simulink model "CAVE_MachE_sil_test_v2"  (R2019b)
settings: configuration reference "ConfigSetDesktopFixedStep" (kept outside this file)
PreLoadFcn:
  | VSS_BICYCLE=Simulink.Variant('Dual=0');
  | VSS_DUAL=Simulink.Variant('Dual=1');
  | Dual=1;
  | load('DriveCycle2.mat')
PostLoadFcn:
  | %if any(exist('dsrtsu_mdlpostloadfcn', 'file') ~= 0), dsrtsu_mdlpostloadfcn('Execute', bdroot); end
InitFcn:
  | , if any(exist('dsmpb_private', 'file') ~= 0), dsmpb_private('dsmpb_mdlclblib', 'Init', bdroot); end,
  | load('DriveCycle2.mat')
model workspace (MAT data in the model file):
  Gas = 0.383333333333
values from neighbouring files (symbols this model uses):
  TestScnrioCycleNum = obj.getParamValue('TestScnrioCycleNum')    [ExpRefBlkCtrl.m]
undefined symbols (not defined in the file or in its folder): AccelCmd, ActTqLF_Nm_, ActTqLR_Nm_, ActTqRF_Nm_, ActTqRR_Nm_, BattChargeLimitMaxPwr, BattChargeLimitSocBpts, BattChargeLimitTbl, BattChrgCapcty, BattDischargeLimitSocBpts, BattDischargeLimitTbl, BattDischargeMaxPwr, BattNumCellsParallel, BattNumCellsSeries, BattOpenVoltCapBpts, BattOpenVoltTbl, BattResistSocBpts, BattResistTbl, BattResistTempBpts, BrakeMaxPrs, BrakeMaxTrq, ChassisDistCg2FrontAxle, ChassisDistCg2RearAxle, ChassisVehMass, CltchCmd, DecelCmd, DiffRatio, EnvGravCnst, EnvPrs, EnvTemp, FuelSpecificGrav, GearCmd, h, InitStates, lgSw, MtrEffSpdBpts, MtrEffTbl, MtrEffTrqBpts, MtrPwrMax, MtrTrqMax, RealSimPara, SteeringCmd, SupvsryCtrlRegenBrkCutOffTbl, SupvsryCtrlRegenSpdBpts, VEH
libraries: vehdynlibtire x8, vehdynlibsuspension x7, vehdynlibtirecommon x7, autolibshared x6, simulink x6, autolibutils x5, VsrLibWheel x4, autolibpowerinfoutils x3, sharedtransform x3, autolibbatterycommon x2, autolibsharedcoupling x2, autolibmappedmotor x2
(part 5 of 10)

== system CAVE_MachE_sil_test_v2/Vehicle Under Test/Vehicle/Vehicle Dynamics/Vehicle 14DOF/Wheels and Tires/VDBS ==
  WheelAng : Inport
  CamberAng : Inport  Port=2  Unit=rad
  AxleTrq : Inport  Port=3
  BrkPrs : Inport  Port=4
  Fz : Inport  Port=5  Unit=N
  r : Inport  Port=6
  VehVel : Inport  Port=7
  Ground Level : Inport  Port=8
  Friction : Inport  Port=9  Unit=1  PortDimensions=4
  Pressure : vehdynlibtirecommon/Constant  const=220000  numWheels=4
      settings: SourceProductName=Vehicle Dynamics Blockset  SourceProductBaseCode=VE
  Terminator : Terminator
  Tire2Veh : Subsystem
  Tires : Subsystem  VariantControlMode=Label  Variant=on  VariantControl=Variant1  LabelModeActiveChoice=0
  Veh2Tire : Subsystem
  scale factors with friction : Subsystem  mask{numWheels=4}
      mask prompts: numWheels "Number of wheels"
  Wheels : Outport  VectorParamsAs1DForOutWhenUnconnected=off
  FrntAxlF : Outport  Port=2  Unit=N  VectorParamsAs1DForOutWhenUnconnected=off
  RearAxlF : Outport  Port=3  Unit=N  VectorParamsAs1DForOutWhenUnconnected=off
  Omega : Outport  Port=4  VectorParamsAs1DForOutWhenUnconnected=off
  Mz : Outport  Port=5  Unit=N*m  VectorParamsAs1DForOutWhenUnconnected=off
  SuspWhlPz : Outport  Port=6  VectorParamsAs1DForOutWhenUnconnected=off
  SuspWhlVz : Outport  Port=7  VectorParamsAs1DForOutWhenUnconnected=off
  wires:
  Ground Level/1 -> Tires/9("Gnd ")
  Pressure/1 -> Tires/7("Press ")
  scale factors with friction/1(lambdas) -> Tires/8("lambda ")
  Fz/1 -> Tires/10("FzSusp "), Tire2Veh/2(Fz)
  AxleTrq/1 -> Veh2Tire/2(Axle)
  BrkPrs/1 -> Veh2Tire/3(Brake)
  VehVel/1 -> Veh2Tire/4(VehVel)
  Veh2Tire/1(T) -> Tires/1("DriveTorque ")
  Veh2Tire/2(P) -> Tires/2("Brake Pressure ")
  Veh2Tire/4(xdotAxle) -> Tires/4("Vx ")
  Veh2Tire/5(ydotAxle) -> Tires/5("Vy ")
  Veh2Tire/3(psidot) -> Tires/3("r ")
  Tires/1(" Wheels") -> Tire2Veh/1(Wheel)
  WheelAng/1 -> Veh2Tire/5(WheelSteer), Tire2Veh/4(WheelSteer)
  Tire2Veh/2(Omega) -> Omega/1
  Tire2Veh/3(FrntAxlF) -> FrntAxlF/1
  Tire2Veh/4(RearAxlF) -> RearAxlF/1
  Tire2Veh/5(<Mz>) -> Mz/1
  Friction/1 -> scale factors with friction/1(lamda_mu_x), scale factors with friction/2(lamda_mu_y)
  r/1 -> Veh2Tire/1(r)
  Veh2Tire/6(zdotAxle) -> Terminator/1
  Tire2Veh/6(SuspWhlPz) -> SuspWhlPz/1
  Tire2Veh/7(SuspWhlVz) -> SuspWhlVz/1
  CamberAng/1 -> Tires/6("Camber "), Tire2Veh/3(WheelCamber), Veh2Tire/6(WheelCamber)
  Tire2Veh/1(Wheels) -> Wheels/1

== system CAVE_MachE_sil_test_v2/Vehicle Under Test/Vehicle/Vehicle Dynamics/Vehicle 7DOF/Longitudinal Wheels 4DOF/Axle Forces ==
  note: 1) Add Subsystem or Model blocks as valid variant choices.
      | 2) You cannot connect blocks at this level. At simulation, connectivity is automatically
      | determined, based on the active variant and port name matching.
  F : Inport
  R : Inport  Port=2
  Bicycle : Subsystem  VariantControl=0
  Dual : Subsystem  VariantControl=1
  FrntAxlF : Outport  Unit=N  VectorParamsAs1DForOutWhenUnconnected=off
  RearAxlF : Outport  Port=2  Unit=N  VectorParamsAs1DForOutWhenUnconnected=off

== system CAVE_MachE_sil_test_v2/Vehicle Under Test/Vehicle/Vehicle Dynamics/Vehicle 7DOF/Longitudinal Wheels 4DOF/Tire2Veh ==
  Wheel : Inport
  Bus Selector7 : BusSelector  OutputSignals=Omega,Fx,Re,z,zdot,Kappa,Alpha
  Dead Zone2 : DeadZone  LowerValue=-5  UpperValue=5  ZeroCross=off  SaturateOnIntegerOverflow=on
  Demux : Demux  Outputs=[2,2]
  Re : Terminator
  Unary Minus1 : UnaryMinus
  Unary Minus2 : UnaryMinus
  zdot : Terminator
  FwF : Outport  VectorParamsAs1DForOutWhenUnconnected=off
  FwR : Outport  Port=2  VectorParamsAs1DForOutWhenUnconnected=off
  z : Outport  Port=3  VectorParamsAs1DForOutWhenUnconnected=off
  Omega : Outport  Port=4  VectorParamsAs1DForOutWhenUnconnected=off
  Kappa : Outport  Port=5  VectorParamsAs1DForOutWhenUnconnected=off
  Alpha : Outport  Port=6  VectorParamsAs1DForOutWhenUnconnected=off
  wires:
  Bus Selector7/2 -> Dead Zone2/1  "<Fx>"
  Dead Zone2/1 -> Demux/1  "Fx"
  Demux/1 -> FwF/1
  Wheel/1 -> Bus Selector7/1
  Bus Selector7/1 -> Omega/1  "<Omega>"
  Bus Selector7/5 -> Unary Minus2/1  "<zdot>"
  Bus Selector7/4 -> Unary Minus1/1  "<z>"
  Unary Minus1/1 -> z/1  "z"
  Demux/2 -> FwR/1
  Bus Selector7/6 -> Kappa/1  "<Kappa>"
  Unary Minus2/1 -> zdot/1  "zdot"
  Bus Selector7/3 -> Re/1  "<Re>"
  Bus Selector7/7 -> Alpha/1  "<Alpha>"

== system CAVE_MachE_sil_test_v2/Vehicle Under Test/Vehicle/Vehicle Dynamics/Vehicle 7DOF/Longitudinal Wheels 4DOF/Tires ==
  AxlTrq : Inport
  BrkPrs : Inport  Port=2
  Vx : Inport  Port=3
  Vy : Inport  Port=4
  r : Inport  Port=5
  Camber : Inport  Port=6
  TirePrs : Inport  Port=7
  Fz : Inport  Port=8
  lam_mu : Inport  Port=9
  Gnd : Inport  Port=10
  4-by-1 Gnd : Subsystem
  4-by-1 Gnd1 : Subsystem
  4-by-1 Gnd2 : Subsystem
  4-by-1 Gnd3 : Subsystem
  Bus Creator : BusCreator  Inputs=12
  Subsystem : Subsystem
  Terminator1 : Terminator
  Terminator2 : Terminator
  Terminator3 : Terminator
  Wheel : Outport  VectorParamsAs1DForOutWhenUnconnected=off
  wires:
  Vy/1 -> Terminator1/1
  Camber/1 -> Terminator2/1
  r/1 -> Terminator3/1
  Bus Creator/1 -> Wheel/1
  Subsystem/7(zdot) -> Bus Creator/10  "zdot"
  Subsystem/6(z) -> Bus Creator/9  "z"
  Subsystem/2(Fx) -> Bus Creator/2  "Fx"
  Subsystem/1(Omega) -> Bus Creator/1  "Omega"
  Subsystem/5(Re) -> Bus Creator/8  "Re"
  Subsystem/3(FzOut) -> Bus Creator/4  "Fz"
  Subsystem/4(My) -> Bus Creator/6  "My"
  4-by-1 Gnd/1(Gnd) -> Bus Creator/3  "Fy"
  4-by-1 Gnd1/1(Gnd) -> Bus Creator/5  "Mx"
  4-by-1 Gnd2/1(Gnd) -> Bus Creator/7  "Mz"
  Subsystem/8(Kappa) -> Bus Creator/11  "Kappa"
  4-by-1 Gnd3/1(Gnd) -> Bus Creator/12  "Alpha"
  AxlTrq/1 -> Subsystem/1(AxlTrq)
  BrkPrs/1 -> Subsystem/2(BrkPrs)
  Vx/1 -> Subsystem/3(Vx)
  TirePrs/1 -> Subsystem/4(TirePrs)
  Fz/1 -> Subsystem/5(Fz)
  lam_mu/1 -> Subsystem/6(lam_mu)
  Gnd/1 -> Subsystem/7(Gnd)

== system CAVE_MachE_sil_test_v2/Vehicle Under Test/Vehicle/Vehicle Dynamics/Vehicle 7DOF/Longitudinal Wheels 4DOF/Veh2Tire ==
  AxlTrq : Inport
  BrkPrs : Inport  Port=2
  r : Inport  Port=3
  VehVel : Inport  Port=4
  WhlAng : Inport  Port=5
  Reshape3 : Reshape
  Reshape4 : Reshape
  Unary Minus : UnaryMinus
  Wheel to Body Transform : Subsystem
  T : Outport  VectorParamsAs1DForOutWhenUnconnected=off
  P : Outport  Port=2  VectorParamsAs1DForOutWhenUnconnected=off
  xdotAxle : Outport  Port=3  VectorParamsAs1DForOutWhenUnconnected=off
  ydotAxle : Outport  Port=4  VectorParamsAs1DForOutWhenUnconnected=off
  psidot : Outport  Port=5  VectorParamsAs1DForOutWhenUnconnected=off
  zdotAxle : Outport  Port=6  VectorParamsAs1DForOutWhenUnconnected=off
  wires:
  BrkPrs/1 -> Reshape3/1
  AxlTrq/1 -> Reshape4/1
  Wheel to Body Transform/1(xdotWheel) -> xdotAxle/1  "Vx"
  Wheel to Body Transform/2(ydotWheel) -> ydotAxle/1  "Vy"
  r/1 -> Unary Minus/1
  Reshape4/1 -> T/1
  VehVel/1 -> Wheel to Body Transform/1(VelVeh)
  WhlAng/1 -> Wheel to Body Transform/2(WhlAng)
  Wheel to Body Transform/3(zdotWheel) -> zdotAxle/1  "Vz"
  Unary Minus/1 -> psidot/1
  Reshape3/1 -> P/1

== system CAVE_MachE_sil_test_v2/Vehicle Under Test/Vehicle/Vehicle Dynamics/Vehicle 7DOF/Longitudinal Wheels 4DOF/Velocity and Vertical Load ==
  note: 1) Add Subsystem or Model blocks as valid variant choices.
      | 2) You cannot connect blocks at this level. At simulation, connectivity is automatically
      | determined, based on the active variant and port name matching.
  VehFdbk : Inport
  Bicycle : Subsystem  VariantControl=0
  Dual : Subsystem  VariantControl=1
  VehVel : Outport  VectorParamsAs1DForOutWhenUnconnected=off
  Fz : Outport  Port=2  PortDimensions=4  VectorParamsAs1DForOutWhenUnconnected=off

== system CAVE_MachE_sil_test_v2/Vehicle Under Test/Vehicle/Vehicle Dynamics/Vehicle 7DOF/Longitudinal Wheels 4DOF/Wheel Angles ==
  WheelAng : Inport
  Camber : Inport  Port=2
  Add1 : Sum
  Constant2 : Constant  Value=0
  Constant3 : Constant  Value=ones(1,4).*pi
  Demux : Demux  Outputs=2
  Demux1 : Demux
  Mux : Mux  Inputs=2
  Reshape : Reshape  OutputDimensionality=Row vector (2-D)
  Reshape1 : Reshape  OutputDimensionality=Row vector (2-D)
  Reshape2 : Reshape  OutputDimensionality=Row vector (2-D)
  Vector Concatenate3 : Concatenate  NumInputs=3  Mode=Multidimensional array
  Vector Concatenate4 : Concatenate  NumInputs=4
  WhlAngB : Outport  VectorParamsAs1DForOutWhenUnconnected=off
  wires:
  Demux1/2 -> Mux/1
  Constant2/1 -> Add1/2
  Add1/1 -> Demux/1
  Demux1/3 -> Vector Concatenate4/3
  Demux1/1 -> Vector Concatenate4/1
  Mux/1 -> Add1/1
  Demux1/4 -> Mux/2
  Demux/1 -> Vector Concatenate4/2
  Demux/2 -> Vector Concatenate4/4
  Vector Concatenate4/1 -> Reshape/1
  Constant3/1 -> Reshape1/1
  Vector Concatenate3/1 -> WhlAngB/1
  Reshape/1 -> Vector Concatenate3/3
  Reshape1/1 -> Vector Concatenate3/1
  Reshape2/1 -> Vector Concatenate3/2
  Camber/1 -> Reshape2/1
  WheelAng/1 -> Demux1/1

== system CAVE_MachE_sil_test_v2/Vehicle Under Test/Vehicle/Vehicle Dynamics/Vehicle 7DOF/Subsystem4/Subsystem ==
  CgXYZdot : Inport
  angles : Inport  Port=2
  Demux2 : Demux  Outputs=3
  Demux3 : Demux  Outputs=3
  Terminator{,1..4} (5 alike) : Terminator
  VehSpd : Outport
  wires:
  CgXYZdot/1 -> Demux2/1
  Demux3/2 -> Terminator3/1  "theta"
  Demux2/2 -> Terminator/1  "Ydot"
  Demux3/1 -> Terminator2/1  "phi"
  Demux3/3 -> Terminator4/1  "psi"
  Demux2/3 -> Terminator1/1  "Zdot"
  angles/1 -> Demux3/1
  Demux2/1 -> VehSpd/1  "Xdot"

== system CAVE_MachE_sil_test_v2/Vehicle Under Test/Vehicle/Vehicle Dynamics/Vehicle 7DOF/Vehicle Body 3DOF External Longitudinal Wheels/Bicycle ==
  WhlAng : Inport
  "FwF " : Inport  Port=2
  "FwR " : Inport  Port=3
  WindXYZ : Inport  Port=4
  Friction : Inport  Port=5
  Demux : Demux  Outputs=[2,2]
  Gain : Gain  Gain=.5
  Gain1 : Gain  Gain=.5
  Gain2 : Gain  Gain=.5
  Selector : Selector  InputPortWidth=4  IndexOptions=Index vector (dialog)  Indices=[1 2]  OutputSizes=1
  Signal Specification : SignalSpecification  Unit=1
  Signal Specification1 : SignalSpecification  Unit=rad
  Sum of Elements : Sum  Inputs=+
  Sum of Elements1 : Sum  Inputs=+
  Sum of Elements2 : Sum  Inputs=+
  Terminator{,1..5} (6 alike) : Terminator
  Vector Concatenate : Concatenate
  Vehicle Body 3DOF Single Track : autolibshared/Vehicle Body 3DOF Single Track  trackMode=Single (bicycle)  inputMode=External longitudinal forces  frontSteerMode=on  rearSteerMode=off  windMode=on  muMode=on  extFMode=off  extMMode=off  extXo=off  extpsio=off  extxdoto=off  extro=off  extYo=off  extTamb=off  extydoto=off  aMode=2  NF=ChassisNumFrontWhls  NR=ChassisNumRearWhls  m=ChassisVehMass  a=ChassisDistCg2FrontAxle  b=ChassisDistCg2RearAxle  h=ChassisCgHeight  X_o=0  xdot_o=20  CalphaMode=off  sigmaMode=on  d=0  w=1.922.*[1 1]  Cy_f=15000  Cy_r=35000  sigma_f=.1  sigma_r=.1  alpha_f_brk=[-.1 .1]  Cy_f_data=[-9e3 9e3]  alpha_r_brk=[-.1 .1]  Cy_r_data=[-9e3 9e3]  Y_o=0  ydot_o=0  Izz=2500  psi_o=0  r_o=0  Af=ChassisFrontalArea  Cd=ChassisDragCoeff  Cl=.1  Cpm=.1  beta_w=[0:0.01:0.3]  Cs=[0:0.03:0.9]  Cym=[0:0.01:0.3]  Pabs=EnvPrs  Tair=EnvTemp  g=EnvGravCnst  mu=1  xdot_tol=1  Fznom=5000  Fxtire_sat=7e3*1e3  Fytire_sat=2e3*1e3  longOff=0  latOff=0  vertOff=.0112  wrapAng=off
      settings: SourceProductName=Powertrain Blockset  SourceProductBaseCode=PW
  Wheel Positions : Subsystem
  " Info" : Outport  VectorParamsAs1DForOutWhenUnconnected=off
  XWheel : Outport  Port=2  Unit=m  VectorParamsAs1DForOutWhenUnconnected=off
  " YWheel" : Outport  Port=3  Unit=m  VectorParamsAs1DForOutWhenUnconnected=off
  wires:
  "FwR "/1 -> Vehicle Body 3DOF Single Track/3
  "FwF "/1 -> Vehicle Body 3DOF Single Track/2
  Vehicle Body 3DOF Single Track/1 -> " Info"/1, Wheel Positions/1(Info)
  WhlAng/1 -> Selector/1
  Gain/1 -> Signal Specification1/1
  Sum of Elements/1 -> Gain/1
  Vehicle Body 3DOF Single Track/6 -> Terminator/1
  Vehicle Body 3DOF Single Track/7 -> Terminator1/1
  WindXYZ/1 -> ?
  Selector/1 -> Sum of Elements/1
  Demux/1 -> Sum of Elements1/1
  Friction/1 -> Demux/1
  Sum of Elements1/1 -> Gain1/1
  Sum of Elements2/1 -> Gain2/1
  Demux/2 -> Sum of Elements2/1
  Gain1/1 -> Vector Concatenate/1
  Gain2/1 -> Vector Concatenate/2
  Vector Concatenate/1 -> Signal Specification/1
  Signal Specification/1 -> ?
  Signal Specification1/1 -> Vehicle Body 3DOF Single Track/1
  Wheel Positions/2(YWheel) -> " YWheel"/1
  Wheel Positions/1(XWheel) -> XWheel/1
  Vehicle Body 3DOF Single Track/4 -> Terminator2/1
  Vehicle Body 3DOF Single Track/5 -> Terminator3/1
  Vehicle Body 3DOF Single Track/2 -> Terminator4/1
  Vehicle Body 3DOF Single Track/3 -> Terminator5/1

== system CAVE_MachE_sil_test_v2/Vehicle Under Test/Vehicle/Vehicle Dynamics/Vehicle 7DOF/Vehicle Body 3DOF External Longitudinal Wheels/Dual ==
  WhlAng : Inport
  "FwF " : Inport  Port=2
  "FwR " : Inport  Port=3
  WindXYZ : Inport  Port=4
  Friction : Inport  Port=5
  Reshape : Reshape  OutputDimensionality=Customize  OutputDimensions=[2,2]
  Selector : Selector  InputPortWidth=4  IndexOptions=Index vector (dialog)  Indices=[1 2]  OutputSizes=1
  Signal Specification : SignalSpecification  Unit=1
  Terminator{,1..5} (6 alike) : Terminator
  Vehicle Body 3DOF Dual Track : autolibshared/Vehicle Body 3DOF Single Track  trackMode=Dual  inputMode=External longitudinal forces  frontSteerMode=on  rearSteerMode=off  windMode=on  muMode=on  extFMode=off  extMMode=off  extXo=off  extpsio=off  extxdoto=off  extro=off  extYo=off  extTamb=off  extydoto=off  aMode=2  NF=ChassisNumFrontWhls  NR=ChassisNumRearWhls  m=ChassisVehMass  a=ChassisDistCg2FrontAxle  b=ChassisDistCg2RearAxle  h=ChassisCgHeight  X_o=0  xdot_o=InitStates(TestScnrioCycleNum).VehSpd  CalphaMode=off  sigmaMode=on  d=0  w=1.9.*[1 1]  Cy_f=15000  Cy_r=35000  sigma_f=.1  sigma_r=.1  alpha_f_brk=[-.1 .1]  Cy_f_data=[-9e3 9e3]  alpha_r_brk=[-.1 .1]  Cy_r_data=[-9e3 9e3]  Y_o=0  ydot_o=0  Izz=2500  psi_o=0  r_o=0  Af=ChassisFrontalArea  Cd=ChassisDragCoeff  Cl=.1  Cpm=.1  beta_w=[0:0.01:0.3]  Cs=[0:0.03:0.9]  Cym=[0:0.01:0.3]  Pabs=EnvPrs  Tair=EnvTemp  g=EnvGravCnst  mu=1  xdot_tol=1  Fznom=5000  Fxtire_sat=7e3*1e3  Fytire_sat=2e3*1e3  longOff=0  latOff=0  vertOff=.0112  wrapAng=off
      settings: SourceProductName=Powertrain Blockset  SourceProductBaseCode=PW
  Wheel Positions : Subsystem
  " Info" : Outport  VectorParamsAs1DForOutWhenUnconnected=off
  " XWheel" : Outport  Port=2  VectorParamsAs1DForOutWhenUnconnected=off
  " YWheel" : Outport  Port=3  VectorParamsAs1DForOutWhenUnconnected=off
  wires:
  WhlAng/1 -> Selector/1
  Selector/1 -> Vehicle Body 3DOF Dual Track/1
  Friction/1 -> Reshape/1
  Reshape/1 -> Signal Specification/1
  Vehicle Body 3DOF Dual Track/1 -> " Info"/1, Wheel Positions/1(Info)
  Wheel Positions/1(XWheel) -> " XWheel"/1
  Wheel Positions/2(YWheel) -> " YWheel"/1
  Vehicle Body 3DOF Dual Track/2 -> Terminator4/1
  Vehicle Body 3DOF Dual Track/3 -> Terminator5/1
  Vehicle Body 3DOF Dual Track/6 -> Terminator1/1
  Vehicle Body 3DOF Dual Track/4 -> Terminator2/1
  Vehicle Body 3DOF Dual Track/5 -> Terminator3/1
  Vehicle Body 3DOF Dual Track/7 -> Terminator/1
  Signal Specification/1 -> ?
  WindXYZ/1 -> ?
  "FwF "/1 -> Vehicle Body 3DOF Dual Track/2
  "FwR "/1 -> Vehicle Body 3DOF Dual Track/3

== system CAVE_MachE_sil_test_v2/Vehicle Under Test/Vehicle/Vehicle Dynamics/Vehicle Longitudinal/Longitudinal Wheels/Front Diff Wheels ==
  BrkPrs : Inport
  AxleTorq : Inport  Port=2
  Add2 : Sum
  Bus Creator : BusCreator  Inputs=3
  Bus Creator5 : BusCreator  Inputs=1
  Bus Selector6 : BusSelector  OutputSignals=VehSpd,FrcZ
  Bus Selector7 : BusSelector  OutputSignals=VehSpd,FrcZ
  Selector : Selector  InputPortWidth=4  IndexOptions=Index vector (dialog)  Indices=1  OutputSizes=1
  Selector1 : Selector  InputPortWidth=4  IndexOptions=Index vector (dialog)  Indices=2  OutputSizes=1
  Selector2 : Selector  InputPortWidth=4  IndexOptions=Index vector (dialog)  Indices=1  OutputSizes=1
  Selector3 : Selector  InputPortWidth=4  IndexOptions=Index vector (dialog)  Indices=2  OutputSizes=1
  Simple Longitudinal Wheel 1 : VsrLibWheel/Simple Longitudinal Wheel  TireLoadedRadius=WhlRearLoadedRadius  C_rr=WhlRollingResistCnst  MaxBrkTrq=BrakeMaxTrq  MaxBrkPrs=BrakeMaxPrs  w_thresh=WhlSimVelTol
  Simple Longitudinal Wheel 2 : VsrLibWheel/Simple Longitudinal Wheel  TireLoadedRadius=WhlRearLoadedRadius  C_rr=WhlRollingResistCnst  MaxBrkTrq=BrakeMaxTrq  MaxBrkPrs=BrakeMaxPrs  w_thresh=WhlSimVelTol
  Terminator3 : Terminator
  Two-Way Connection6 : TwoWayConnection
  DiffAxle : PMIOPort  Side=Right
  Info : Outport
  wires:
  Bus Selector6/2 -> Simple Longitudinal Wheel 1/4  "<FrcZ>"
  BrkPrs/1 -> Selector3/1, Selector2/1
  Simple Longitudinal Wheel 1/2 -> Add2/1
  Bus Selector7/1 -> Simple Longitudinal Wheel 2/3  "<VehSpd>"
  Bus Selector6/1 -> Simple Longitudinal Wheel 1/3  "<VehSpd>"
  Bus Selector7/2 -> Simple Longitudinal Wheel 2/4  "<FrcZ>"
  Two-Way Connection6/1 -> Bus Selector7/1, Bus Selector6/1
  Add2/1 -> Bus Creator5/1  "FrcX"
  Simple Longitudinal Wheel 2/2 -> Add2/2  "Spd"
  Bus Creator5/1 -> Two-Way Connection6/1
  Simple Longitudinal Wheel 2/1 -> Terminator3/1
  Selector2/1 -> Simple Longitudinal Wheel 1/1
  AxleTorq/1 -> Selector1/1, Selector/1
  Selector/1 -> Simple Longitudinal Wheel 1/2
  Selector1/1 -> Simple Longitudinal Wheel 2/2
  Selector3/1 -> Simple Longitudinal Wheel 2/1
  Simple Longitudinal Wheel 1/3 -> Bus Creator/2  "Omega1"
  Bus Creator/1 -> Info/1
  Simple Longitudinal Wheel 1/1 -> Bus Creator/1  "WhlFrontInfo"
  Simple Longitudinal Wheel 2/3 -> Bus Creator/3  "Omega2"
  connections:
  DiffAxle/RConn1 -- Two-Way Connection6/RConn1

== system CAVE_MachE_sil_test_v2/Vehicle Under Test/Vehicle/Vehicle Dynamics/Vehicle Longitudinal/Longitudinal Wheels/Rear Wheels ==
  BrkPrs : Inport
  Add2 : Sum
  Bus Creator : BusCreator  Inputs=3
  Bus Creator5 : BusCreator  Inputs=1
  Bus Selector6 : BusSelector  OutputSignals=VehSpd,FrcZ
  Bus Selector7 : BusSelector  OutputSignals=VehSpd,FrcZ
  Ground : Ground
  Selector : Selector  InputPortWidth=4  IndexOptions=Index vector (dialog)  Indices=3  OutputSizes=1
  Selector1 : Selector  InputPortWidth=4  IndexOptions=Index vector (dialog)  Indices=4  OutputSizes=1
  Simple Longitudinal Wheel : VsrLibWheel/Simple Longitudinal Wheel  TireLoadedRadius=WhlFrontLoadedRadius  C_rr=WhlRollingResistCnst  MaxBrkTrq=BrakeMaxTrq  MaxBrkPrs=BrakeMaxPrs  w_thresh=WhlSimVelTol
  Simple Longitudinal Wheel1 : VsrLibWheel/Simple Longitudinal Wheel  TireLoadedRadius=WhlFrontLoadedRadius  C_rr=WhlRollingResistCnst  MaxBrkTrq=BrakeMaxTrq  MaxBrkPrs=BrakeMaxPrs  w_thresh=WhlSimVelTol
  Terminator3 : Terminator
  Two-Way Connection6 : TwoWayConnection
  DiffAxle : PMIOPort  Side=Right
  Info : Outport
  wires:
  Simple Longitudinal Wheel1/1 -> Terminator3/1
  Simple Longitudinal Wheel1/3 -> Bus Creator/3  "Omega4"
  Ground/1 -> Simple Longitudinal Wheel/2, Simple Longitudinal Wheel1/2
  Simple Longitudinal Wheel/3 -> Bus Creator/2  "Omega3"
  Bus Creator5/1 -> Two-Way Connection6/1
  Simple Longitudinal Wheel1/2 -> Add2/2  "Spd"
  Add2/1 -> Bus Creator5/1  "FrcX"
  Two-Way Connection6/1 -> Bus Selector7/1, Bus Selector6/1
  Bus Selector7/2 -> Simple Longitudinal Wheel1/4  "<FrcZ>"
  Bus Selector6/1 -> Simple Longitudinal Wheel/3  "<VehSpd>"
  Bus Selector7/1 -> Simple Longitudinal Wheel1/3  "<VehSpd>"
  Simple Longitudinal Wheel/2 -> Add2/1
  BrkPrs/1 -> Selector1/1, Selector/1
  Bus Selector6/2 -> Simple Longitudinal Wheel/4  "<FrcZ>"
  Selector/1 -> Simple Longitudinal Wheel/1
  Selector1/1 -> Simple Longitudinal Wheel1/1
  Simple Longitudinal Wheel/1 -> Bus Creator/1  "WhlRearInfo"
  Bus Creator/1 -> Info/1
  connections:
  DiffAxle/RConn1 -- Two-Way Connection6/RConn1

== system CAVE_MachE_sil_test_v2/Vehicle Under Test/Vehicle/Vehicle Dynamics/Vehicle Longitudinal/Vehicle Body/Logitudinal Vehicle Body ==
  RoadGrade : Inport
  WindVel : Inport  Port=2  Unit=m/s
  Bus Creator : BusCreator  Inputs=2
  Bus Creator1 : BusCreator  Inputs=2
  Bus Selector : BusSelector  OutputSignals=FrcX
  Bus Selector1 : BusSelector  OutputSignals=BdyFrm.Cg.Vel.xdot,BdyFrm.Cg.Disp.x
  Bus Selector3 : BusSelector  OutputSignals=FrcX
  Signal Specification3 : SignalSpecification  Unit=N
  Signal Specification4 : SignalSpecification  Unit=N
  Transfer Fcn : TransferFcn  Denominator=[0.01 1]
  Transfer Fcn1 : TransferFcn  Denominator=[0.01 1]
  Two-Way Connection2 : TwoWayConnection
  Two-Way Connection8 : TwoWayConnection
  Unit Conversion : UnitConversion
  Vehicle Body 1DOF Longitudinal : autolibshared/Vehicle Body 1DOF Longitudinal  VariantControl=SL  extFMode=off  extMMode=off  extTamb=off  wind3D=off  aMode=1  NF=ChassisNumFrontWhls  NR=ChassisNumRearWhls  m=ChassisVehMass  a=ChassisDistCg2FrontAxle  b=ChassisDistCg2RearAxle  h=ChassisCgHeight  Cd=ChassisDragCoeff  Cl=0  Cpm=0  Af=ChassisFrontalArea  x_o=0  xdot_o=InitStates(TestScnrioCycleNum).VehSpd  Pabs=EnvPrs  T=EnvTemp  g=EnvGravCnst
      settings: SourceProductName=Powertrain Blockset  SourceProductBaseCode=PW
  Front : PMIOPort  Side=Left
  Rear : PMIOPort  Port=2  Side=Left
  VehSpd : Outport  VectorParamsAs1DForOutWhenUnconnected=off
  VehDist : Outport  Port=2  VectorParamsAs1DForOutWhenUnconnected=off
  FrontAxleFrc : Outport  Port=3  VectorParamsAs1DForOutWhenUnconnected=off
  RearAxleFrc : Outport  Port=4  VectorParamsAs1DForOutWhenUnconnected=off
  wires:
  Two-Way Connection8/1 -> Bus Selector/1
  RoadGrade/1 -> Unit Conversion/1
  Bus Selector/1 -> Transfer Fcn1/1  "<FrcX>"
  Vehicle Body 1DOF Longitudinal/2 -> Bus Creator/1, Bus Creator1/1  "VehSpd"
  Vehicle Body 1DOF Longitudinal/1 -> Bus Selector1/1  "Veh"
  Signal Specification3/1 -> RearAxleFrc/1, Vehicle Body 1DOF Longitudinal/2  "RearAxleFrc"
  Bus Creator/1 -> Two-Way Connection8/1
  Vehicle Body 1DOF Longitudinal/3 -> Bus Creator/2  "FrcZ"
  WindVel/1 -> Vehicle Body 1DOF Longitudinal/4
  Two-Way Connection2/1 -> Bus Selector3/1
  Vehicle Body 1DOF Longitudinal/4 -> Bus Creator1/2  "FrcZ"
  Bus Selector1/1 -> VehSpd/1  "<xdot>"
  Bus Selector1/2 -> VehDist/1  "<x>"
  Unit Conversion/1 -> Vehicle Body 1DOF Longitudinal/3
  Signal Specification4/1 -> FrontAxleFrc/1, Vehicle Body 1DOF Longitudinal/1  "FrontAxleFrc"
  Transfer Fcn/1 -> Signal Specification3/1
  Transfer Fcn1/1 -> Signal Specification4/1
  Bus Creator1/1 -> Two-Way Connection2/1
  Bus Selector3/1 -> Transfer Fcn/1  "<FrcX>"
  connections:
  Two-Way Connection8/RConn1 -- Front/RConn1
  Two-Way Connection2/RConn1 -- Rear/RConn1

== system CAVE_MachE_sil_test_v2/Vehicle Under Test/Vehicle/Vehicle Dynamics/Vehicle Longitudinal/Vehicle Body/Subsystem1 ==
  VehSpd : Inport
  VehDist : Inport  Port=2
  FrontAxleFrc : Inport  Port=3
  RearAxleFrc : Inport  Port=4
  Bus Creator : BusCreator  Inputs=4
  ChassisPlant : Outport
  wires:
  VehSpd/1 -> Bus Creator/1  "VehSpd"
  VehDist/1 -> Bus Creator/2  "VehDist"
  Bus Creator/1 -> ChassisPlant/1  "ChassisPlant"
  FrontAxleFrc/1 -> Bus Creator/3  "FrontAxleFrc"
  RearAxleFrc/1 -> Bus Creator/4  "RearAxleFrc"

== system CAVE_MachE_sil_test_v2/Vehicle Under Test/Vehicle/Battery/Battery/Lithium Ion Battery Pack1/Datasheet Battery Internal/Datasheet Battery ==
  CapInit : Inport  Unit=A*hr
  BattCurr : Inport  Port=2  Unit=A
  BattTemp : Inport  Port=3  Unit=K
  Charge Model : Subsystem
  State of Charge Capacity : Subsystem
  Voltage and Power Calculation : Subsystem
  LdCurrFeed : Outport  Unit=A  VectorParamsAs1DForOutWhenUnconnected=off
  OutVoltUnfilt : Outport  Port=2  Unit=V  VectorParamsAs1DForOutWhenUnconnected=off
  LdAmpHr : Outport  Port=3  Unit=A*hr  VectorParamsAs1DForOutWhenUnconnected=off
  BattSoc : Outport  Port=4  Unit=1  VectorParamsAs1DForOutWhenUnconnected=off
  BattPwrLoss : Outport  Port=5  Unit=V  VectorParamsAs1DForOutWhenUnconnected=off
  wires:
  Voltage and Power Calculation/2(BattPwrLoss) -> BattPwrLoss/1
  CapInit/1 -> Charge Model/2(CapInit)
  BattTemp/1 -> Voltage and Power Calculation/3(BattTemp)
  State of Charge Capacity/1(CapSOC) -> BattSoc/1, Voltage and Power Calculation/1(CapSOC)
  Charge Model/1(LdAmpHr) -> LdAmpHr/1, State of Charge Capacity/1(LdAmpHr)
  Voltage and Power Calculation/1(OutVolt) -> OutVoltUnfilt/1
  BattCurr/1 -> Charge Model/1(LdAmp), Voltage and Power Calculation/2(LdAmp), LdCurrFeed/1

== system CAVE_MachE_sil_test_v2/Vehicle Under Test/Vehicle/Powertrain Supervisory Controller /Engine Torque Command/Motor Torque Arbitration and Power Management/Power Management/Check Within Limits ==
  up : Inport
  u : Inport  Port=2
  lo : Inport  Port=3
  Compare To Zero : simulink/Logic and Bit Operations/Compare To Zero  relop=>=  OutDataTypeStr=boolean
  Compare To Zero1 : simulink/Logic and Bit Operations/Compare To Zero  relop=<=  OutDataTypeStr=boolean
  Logical Operator : Logic  AllPortsSameDT=off  OutDataTypeStr=boolean
  Saturation Dynamic1 : simulink/Discontinuities/Saturation Dynamic  OutMin=[]  OutMax=[]  OutDataTypeStr=Inherit: Same as second input  OutDataType=fixdt(1, 16)  OutScaling=2^-10  DoSatur=off
  Subtract : Sum  Inputs=+-
  Subtract1 : Sum  Inputs=-+
  InLimit : Outport  VectorParamsAs1DForOutWhenUnconnected=off
  y : Outport  Port=2  VectorParamsAs1DForOutWhenUnconnected=off
  wires:
  Logical Operator/1 -> InLimit/1
  Compare To Zero1/1 -> Logical Operator/2
  Compare To Zero/1 -> Logical Operator/1
  Subtract1/1 -> Compare To Zero1/1
  Subtract/1 -> Compare To Zero/1
  u/1 -> Saturation Dynamic1/2, Subtract/2, Subtract1/1
  up/1 -> Saturation Dynamic1/1, Subtract/1
  lo/1 -> Saturation Dynamic1/3, Subtract1/2
  Saturation Dynamic1/1 -> y/1

== system CAVE_MachE_sil_test_v2/Vehicle Under Test/Vehicle/Powertrain Supervisory Controller /Engine Torque Command/Motor Torque Arbitration and Power Management/Power Management/Mech to Elec Power Estimate ==
  note: Pelec_req = Pmech_req*Eff^k,
      | k = -1 if Motoring >= 0,
      | k = 1 if Generating < 0
  note: Using an Efficiency Map, we can estimate the
      | Electric Power from the Mechanical  Torque Request.
  note: Check if Motoring
      | or Generating
  MotTrqCmd : Inport
  MotSpd : Inport  Port=2
  Abs : Abs
  Abs1 : Abs
  Constant1 : Constant  Value=-1  SampleTime=-1
  Constant2 : Constant  SampleTime=-1
  Eff Map : Lookup_n-D  BreakpointsForDimension1=MtrEffSpdBpts  BreakpointsForDimension2=MtrEffTrqBpts  Table=MtrEffTbl  ExtrapMethod=Clip  UseLastTableValue=on  InternalRulePriority=Speed  OutDataTypeStr=Inherit: Inherit from 'Table data'  RndMeth=Simplest  InputSameDT=on
  Gain1 : Gain  Gain=1/100
  Math Function : Math  Operator=pow  OutputSignalType=real  SaturateOnIntegerOverflow=on
  Product : Product
  Product3 : Product
  Product4 : Product
  Switch2 : Switch
  rads_to_rpm : Gain  Gain=30/pi
  MotPwrElecReq : Outport  VectorParamsAs1DForOutWhenUnconnected=off
  Eff2k : Outport  Port=2  VectorParamsAs1DForOutWhenUnconnected=off
  wires:
  MotTrqCmd/1 -> Abs1/1, Product/2, Product3/2
  MotSpd/1 -> rads_to_rpm/1, Product/1, Product3/1
  Product/1 -> Switch2/2
  rads_to_rpm/1 -> Abs/1
  Abs1/1 -> Eff Map/2
  Product4/1 -> MotPwrElecReq/1
  Math Function/1 -> Product4/2, Eff2k/1
  Gain1/1 -> Math Function/1
  Abs/1 -> Eff Map/1
  Eff Map/1 -> Gain1/1
  Constant2/1 -> Switch2/3
  Constant1/1 -> Switch2/1
  Switch2/1 -> Math Function/2
  Product3/1 -> Product4/1

== system CAVE_MachE_sil_test_v2/Vehicle Under Test/Vehicle/Powertrain Supervisory Controller /Engine Torque Command/Motor Torque Arbitration and Power Management/Power Management/Torque Limit ==
  MotTrq : Inport
  MotSpd : Inport  Port=2
  Gain : Gain  Gain=-1
  Max Motor Torque : LibPtSupervisoryCtrl/Powertrain Supervisory Controller /Engine Torque Command/Accel Pedal to Traction Wheel Torque Request/Max Motor Torque  SystemSampleTime=-1  Latency=0  AutoFrameSizeCalculation=off
  Saturation Dynamic : simulink/Discontinuities/Saturation Dynamic  OutMin=[]  OutMax=[]  OutDataTypeStr=Inherit: Same as second input  OutDataType=fixdt(1, 16)  OutScaling=2^-10  DoSatur=off
  MotTrqCmd : Outport  VectorParamsAs1DForOutWhenUnconnected=off
  wires:
  MotSpd/1 -> Max Motor Torque/1
  Gain/1 -> Saturation Dynamic/3
  Max Motor Torque/1 -> Saturation Dynamic/1, Gain/1
  Saturation Dynamic/1 -> MotTrqCmd/1
  MotTrq/1 -> Saturation Dynamic/2

== system CAVE_MachE_sil_test_v2/Vehicle Under Test/Vehicle/Vehicle Dynamics/Vehicle 14DOF/Suspension/Double Wishbone Suspension/Steer Rate Adapter ==
  Veh : Inport
  Add : Sum
  Bus Selector3 : BusSelector  OutputSignals=BdyFrm.Cg.AngVel.r
  Constant : Constant  Value=zeros(1,4)
  Matrix Concatenate : Concatenate  NumInputs=3  Mode=Multidimensional array
  Matrix Concatenate1 : Concatenate  NumInputs=3  Mode=Multidimensional array
  Reshape2 : Reshape  OutputDimensionality=Row vector (2-D)
  Reshape3 : Reshape  OutputDimensionality=Row vector (2-D)
  Reshape4 : Reshape  OutputDimensionality=Row vector (2-D)
  Selector3 : Selector  InputPortWidth=1  IndexOptions=Index vector (dialog)  Indices=[1 1 1 1]  OutputSizes=1
  SteerRates : Constant  Value=zeros(1,4)
  AngVel : Outport  VectorParamsAs1DForOutWhenUnconnected=off
  wires:
  Reshape2/1 -> Matrix Concatenate1/1, Matrix Concatenate1/3, Matrix Concatenate1/2
  Constant/1 -> Reshape3/1
  Selector3/1 -> Reshape4/1
  Bus Selector3/1 -> Selector3/1  "<r>"
  Matrix Concatenate/1 -> Add/2
  SteerRates/1 -> Reshape2/1
  Reshape4/1 -> Matrix Concatenate/3
  Reshape3/1 -> Matrix Concatenate/2, Matrix Concatenate/1
  Matrix Concatenate1/1 -> Add/1
  Veh/1 -> Bus Selector3/1
  Add/1 -> AngVel/1  "AngVel"

== system CAVE_MachE_sil_test_v2/Vehicle Under Test/Vehicle/Vehicle Dynamics/Vehicle 14DOF/Suspension/Double Wishbone Suspension/Steering Adapter ==
  Steer : Inport
  Reshape1 : Reshape  OutputDimensionality=Row vector (2-D)
  Selector : Selector  IndexOptions=Index vector (dialog)  Indices=[1 2]  OutputSizes=1
  StrgAng : Outport  VectorParamsAs1DForOutWhenUnconnected=off
  wires:
  Reshape1/1 -> StrgAng/1
  Steer/1 -> Selector/1
  Selector/1 -> Reshape1/1

== system CAVE_MachE_sil_test_v2/Vehicle Under Test/Vehicle/Vehicle Dynamics/Vehicle 14DOF/Suspension/Double Wishbone Suspension/Vehicle Adapter ==
  Veh : Inport
  Bus Creator3 : BusCreator  Inputs=2
  Bus Selector1 : BusSelector  OutputSignals=InertFrm.FrntAxl.Lft.Disp.X,InertFrm.FrntAxl.Lft.Disp.Y,InertFrm.FrntAxl.Lft.Disp.Z,InertFrm.FrntAxl.Rght.Disp.X,InertFrm.FrntAxl.Rght.Disp.Y,InertFrm.FrntAxl.Rght.Disp.Z,InertFrm.RearAxl.Lft.Disp.X,InertFrm.RearAxl.Lft.Disp.Y,InertFrm.RearAxl.Lft.Disp.Z,InertFrm.RearAxl.Rght.Disp.X,InertFrm.RearAxl.Rght.Disp.Y,InertFrm.RearAxl.Rght.Disp.Z
  Bus Selector2 : BusSelector  OutputSignals=BdyFrm.FrntAxl.Lft.Vel.xdot,BdyFrm.FrntAxl.Lft.Vel.ydot,BdyFrm.FrntAxl.Lft.Vel.zdot,BdyFrm.FrntAxl.Rght.Vel.xdot,BdyFrm.FrntAxl.Rght.Vel.ydot,BdyFrm.FrntAxl.Rght.Vel.zdot,BdyFrm.RearAxl.Lft.Vel.xdot,BdyFrm.RearAxl.Lft.Vel.ydot,BdyFrm.RearAxl.Lft.Vel.zdot,BdyFrm.RearAxl.Rght.Vel.xdot,BdyFrm.RearAxl.Rght.Vel.ydot,BdyFrm.RearAxl.Rght.Vel.zdot
  Inertial Frame CG to Axle Offset : Constant  Value=[zeros(2,4);h*ones(1,4)+VEH.InitialVertPosition*0]
  Mux1 : Mux  Inputs=12
  Mux2 : Mux  Inputs=12
  Reshape1 : Reshape  OutputDimensionality=Customize  OutputDimensions=[3,4]
  Reshape2 : Reshape  OutputDimensionality=Customize  OutputDimensions=[3,4]
  Sum : Sum  Inputs=|+-
  VehSusp : Outport  VectorParamsAs1DForOutWhenUnconnected=off
  wires:
  Reshape2/1 -> Bus Creator3/2  "V"
  Bus Creator3/1 -> VehSusp/1  "Veh"
  Bus Selector1/1 -> Mux2/1  "<X>"
  Bus Selector1/2 -> Mux2/2  "<Y>"
  Bus Selector1/3 -> Mux2/3  "<Z>"
  Bus Selector1/4 -> Mux2/4  "<X>"
  Bus Selector1/5 -> Mux2/5  "<Y>"
  Bus Selector1/6 -> Mux2/6  "<Z>"
  Bus Selector1/7 -> Mux2/7  "<X>"
  Bus Selector1/8 -> Mux2/8  "<Y>"
  Bus Selector1/9 -> Mux2/9  "<Z>"
  Bus Selector1/10 -> Mux2/10  "<X>"
  Bus Selector1/11 -> Mux2/11  "<Y>"
  Bus Selector1/12 -> Mux2/12  "<Z>"
  Bus Selector2/1 -> Mux1/1  "<xdot>"
  Bus Selector2/2 -> Mux1/2  "<ydot>"
  Bus Selector2/3 -> Mux1/3  "<zdot>"
  Bus Selector2/4 -> Mux1/4  "<xdot>"
  Bus Selector2/5 -> Mux1/5  "<ydot>"
  Bus Selector2/6 -> Mux1/6  "<zdot>"
  Bus Selector2/7 -> Mux1/7  "<xdot>"
  Bus Selector2/8 -> Mux1/8  "<ydot>"
  Bus Selector2/9 -> Mux1/9  "<zdot>"
  Bus Selector2/10 -> Mux1/10  "<xdot>"
  Bus Selector2/11 -> Mux1/11  "<ydot>"
  Bus Selector2/12 -> Mux1/12  "<zdot>"
  Mux1/1 -> Reshape2/1
  Inertial Frame CG to Axle Offset/1 -> Sum/2
  Sum/1 -> Bus Creator3/1  "P"
  Veh/1 -> Bus Selector2/1, Bus Selector1/1
  Mux2/1 -> Reshape1/1
  Reshape1/1 -> Sum/1

== system CAVE_MachE_sil_test_v2/Vehicle Under Test/Vehicle/Vehicle Dynamics/Vehicle 14DOF/Suspension/Double Wishbone Suspension/Wheel  Adapter ==
  Wheels : Inport
  Bus Selector : BusSelector  OutputSignals=TireFrame.Fx,TireFrame.Fy
  Bus Selector1 : BusSelector  OutputSignals=TireFrame.Re
  Bus Selector2 : BusSelector  OutputSignals=TireFrame.Mx,TireFrame.My,TireFrame.Mz
  Bus Selector3 : BusSelector  OutputSignals=TireFrame.z,TireFrame.zdot
  Matrix Concatenate : Concatenate  NumInputs=3  Mode=Multidimensional array
  Reshape{,1..7} (8 alike) : Reshape  OutputDimensionality=Row vector (2-D)
  WhlFx : Outport  VectorParamsAs1DForOutWhenUnconnected=off
  WhlFy : Outport  Port=2  VectorParamsAs1DForOutWhenUnconnected=off
  z : Outport  Port=3  VectorParamsAs1DForOutWhenUnconnected=off
  zdot : Outport  Port=4  VectorParamsAs1DForOutWhenUnconnected=off
  M : Outport  Port=5  VectorParamsAs1DForOutWhenUnconnected=off
  Re : Outport  Port=6  VectorParamsAs1DForOutWhenUnconnected=off
  wires:
  Reshape7/1 -> WhlFy/1
  Reshape6/1 -> WhlFx/1
  Bus Selector/1 -> Reshape6/1  "<Fx>"
  Bus Selector/2 -> Reshape7/1  "<Fy>"
  Bus Selector3/1 -> Reshape/1  "<z>"
  Wheels/1 -> Bus Selector1/1, Bus Selector2/1, Bus Selector3/1, Bus Selector/1
  Bus Selector3/2 -> Reshape2/1  "<zdot>"
  Reshape2/1 -> zdot/1  "zdot"
  Bus Selector1/1 -> Reshape1/1  "<Re>"
  Reshape1/1 -> Re/1  "Re"
  Bus Selector2/1 -> Reshape3/1  "<Mx>"
  Bus Selector2/2 -> Reshape4/1  "<My>"
  Bus Selector2/3 -> Reshape5/1  "<Mz>"
  Reshape3/1 -> Matrix Concatenate/1
  Reshape4/1 -> Matrix Concatenate/2
  Reshape5/1 -> Matrix Concatenate/3
  Matrix Concatenate/1 -> M/1  "M"
  Reshape/1 -> z/1  "z"

== system CAVE_MachE_sil_test_v2/Vehicle Under Test/Vehicle/Vehicle Dynamics/Vehicle 14DOF/Suspension/Independent Mapped Front Suspension Mapped Solid Axle Rear Suspension/Steer Rate Adapter ==
  Veh : Inport
  Add : Sum
  Bus Selector3 : BusSelector  OutputSignals=BdyFrm.Cg.AngVel.r
  Constant : Constant  Value=zeros(1,4)
  Matrix Concatenate : Concatenate  NumInputs=3  Mode=Multidimensional array
  Matrix Concatenate1 : Concatenate  NumInputs=3  Mode=Multidimensional array
  Reshape2 : Reshape  OutputDimensionality=Row vector (2-D)
  Reshape3 : Reshape  OutputDimensionality=Row vector (2-D)
  Reshape4 : Reshape  OutputDimensionality=Row vector (2-D)
  Selector3 : Selector  InputPortWidth=1  IndexOptions=Index vector (dialog)  Indices=[1 1 1 1]  OutputSizes=1
  SteerRates : Constant  Value=zeros(1,4)
  AngVel : Outport  VectorParamsAs1DForOutWhenUnconnected=off
  wires:
  Reshape2/1 -> Matrix Concatenate1/1, Matrix Concatenate1/3, Matrix Concatenate1/2
  Constant/1 -> Reshape3/1
  Selector3/1 -> Reshape4/1
  Bus Selector3/1 -> Selector3/1  "<r>"
  Matrix Concatenate/1 -> Add/2
  SteerRates/1 -> Reshape2/1
  Reshape4/1 -> Matrix Concatenate/3
  Reshape3/1 -> Matrix Concatenate/2, Matrix Concatenate/1
  Matrix Concatenate1/1 -> Add/1
  Veh/1 -> Bus Selector3/1
  Add/1 -> AngVel/1  "AngVel"

== system CAVE_MachE_sil_test_v2/Vehicle Under Test/Vehicle/Vehicle Dynamics/Vehicle 14DOF/Suspension/Independent Mapped Front Suspension Mapped Solid Axle Rear Suspension/Steering Adapter ==
  Steer : Inport
  Reshape1 : Reshape  OutputDimensionality=Row vector (2-D)
  Selector : Selector  IndexOptions=Index vector (dialog)  Indices=[1 2]  OutputSizes=1
  StrgAng : Outport  VectorParamsAs1DForOutWhenUnconnected=off
  wires:
  Reshape1/1 -> StrgAng/1
  Steer/1 -> Selector/1
  Selector/1 -> Reshape1/1

== system CAVE_MachE_sil_test_v2/Vehicle Under Test/Vehicle/Vehicle Dynamics/Vehicle 14DOF/Suspension/Independent Mapped Front Suspension Mapped Solid Axle Rear Suspension/Vehicle Adapter ==
  Veh : Inport
  Bus Creator3 : BusCreator  Inputs=2
  Bus Selector1 : BusSelector  OutputSignals=InertFrm.FrntAxl.Lft.Disp.X,InertFrm.FrntAxl.Lft.Disp.Y,InertFrm.FrntAxl.Lft.Disp.Z,InertFrm.FrntAxl.Rght.Disp.X,InertFrm.FrntAxl.Rght.Disp.Y,InertFrm.FrntAxl.Rght.Disp.Z,InertFrm.RearAxl.Lft.Disp.X,InertFrm.RearAxl.Lft.Disp.Y,InertFrm.RearAxl.Lft.Disp.Z,InertFrm.RearAxl.Rght.Disp.X,InertFrm.RearAxl.Rght.Disp.Y,InertFrm.RearAxl.Rght.Disp.Z
  Bus Selector2 : BusSelector  OutputSignals=BdyFrm.FrntAxl.Lft.Vel.xdot,BdyFrm.FrntAxl.Lft.Vel.ydot,BdyFrm.FrntAxl.Lft.Vel.zdot,BdyFrm.FrntAxl.Rght.Vel.xdot,BdyFrm.FrntAxl.Rght.Vel.ydot,BdyFrm.FrntAxl.Rght.Vel.zdot,BdyFrm.RearAxl.Lft.Vel.xdot,BdyFrm.RearAxl.Lft.Vel.ydot,BdyFrm.RearAxl.Lft.Vel.zdot,BdyFrm.RearAxl.Rght.Vel.xdot,BdyFrm.RearAxl.Rght.Vel.ydot,BdyFrm.RearAxl.Rght.Vel.zdot
  Inertial Frame CG to Axle Offset : Constant  Value=[zeros(2,4);h*ones(1,4)]
  Mux1 : Mux  Inputs=12
  Mux2 : Mux  Inputs=12
  Reshape : Reshape  OutputDimensionality=Customize  OutputDimensions=[3,4]
  Reshape2 : Reshape  OutputDimensionality=Customize  OutputDimensions=[3,4]
  Sum : Sum  Inputs=|+-
  VehSusp : Outport  VectorParamsAs1DForOutWhenUnconnected=off
  wires:
  Veh/1 -> Bus Selector2/1, Bus Selector1/1
  Reshape2/1 -> Bus Creator3/2  "V"
  Bus Creator3/1 -> VehSusp/1  "Veh"
  Reshape/1 -> Sum/1
  Bus Selector1/1 -> Mux2/1  "<X>"
  Bus Selector1/2 -> Mux2/2  "<Y>"
  Bus Selector1/3 -> Mux2/3  "<Z>"
  Bus Selector1/4 -> Mux2/4  "<X>"
  Bus Selector1/5 -> Mux2/5  "<Y>"
  Bus Selector1/6 -> Mux2/6  "<Z>"
  Bus Selector1/7 -> Mux2/7  "<X>"
  Bus Selector1/8 -> Mux2/8  "<Y>"
  Bus Selector1/9 -> Mux2/9  "<Z>"
  Bus Selector1/10 -> Mux2/10  "<X>"
  Bus Selector1/11 -> Mux2/11  "<Y>"
  Bus Selector1/12 -> Mux2/12  "<Z>"
  Bus Selector2/1 -> Mux1/1  "<xdot>"
  Bus Selector2/2 -> Mux1/2  "<ydot>"
  Bus Selector2/3 -> Mux1/3  "<zdot>"
  Bus Selector2/4 -> Mux1/4  "<xdot>"
  Bus Selector2/5 -> Mux1/5  "<ydot>"
  Bus Selector2/6 -> Mux1/6  "<zdot>"
  Bus Selector2/7 -> Mux1/7  "<xdot>"
  Bus Selector2/8 -> Mux1/8  "<ydot>"
  Bus Selector2/9 -> Mux1/9  "<zdot>"
  Bus Selector2/10 -> Mux1/10  "<xdot>"
  Bus Selector2/11 -> Mux1/11  "<ydot>"
  Bus Selector2/12 -> Mux1/12  "<zdot>"
  Mux1/1 -> Reshape2/1
  Mux2/1 -> Reshape/1
  Inertial Frame CG to Axle Offset/1 -> Sum/2
  Sum/1 -> Bus Creator3/1  "P"

== system CAVE_MachE_sil_test_v2/Vehicle Under Test/Vehicle/Vehicle Dynamics/Vehicle 14DOF/Suspension/Independent Mapped Front Suspension Mapped Solid Axle Rear Suspension/Wheel  Adapter ==
  Wheels : Inport
  Bus Selector : BusSelector  OutputSignals=TireFrame.Fx,TireFrame.Fy
  Bus Selector1 : BusSelector  OutputSignals=TireFrame.Re
  Bus Selector2 : BusSelector  OutputSignals=TireFrame.Mx,TireFrame.My,TireFrame.Mz
  Bus Selector3 : BusSelector  OutputSignals=TireFrame.z,TireFrame.zdot
  Matrix Concatenate : Concatenate  NumInputs=3  Mode=Multidimensional array
  Reshape{,1..7} (8 alike) : Reshape  OutputDimensionality=Row vector (2-D)
  WhlFx : Outport  VectorParamsAs1DForOutWhenUnconnected=off
  WhlFy : Outport  Port=2  VectorParamsAs1DForOutWhenUnconnected=off
  z : Outport  Port=3  VectorParamsAs1DForOutWhenUnconnected=off
  zdot : Outport  Port=4  VectorParamsAs1DForOutWhenUnconnected=off
  M : Outport  Port=5  VectorParamsAs1DForOutWhenUnconnected=off
  Re : Outport  Port=6  VectorParamsAs1DForOutWhenUnconnected=off
  wires:
  Reshape7/1 -> WhlFy/1
  Reshape6/1 -> WhlFx/1
  Bus Selector/1 -> Reshape6/1  "<Fx>"
  Bus Selector/2 -> Reshape7/1  "<Fy>"
  Bus Selector3/1 -> Reshape/1  "<z>"
  Wheels/1 -> Bus Selector1/1, Bus Selector2/1, Bus Selector3/1, Bus Selector/1
  Bus Selector3/2 -> Reshape2/1  "<zdot>"
  Reshape2/1 -> zdot/1  "zdot"
  Bus Selector1/1 -> Reshape1/1  "<Re>"
  Reshape1/1 -> Re/1  "Re"
  Bus Selector2/1 -> Reshape3/1  "<Mx>"
  Bus Selector2/2 -> Reshape4/1  "<My>"
  Bus Selector2/3 -> Reshape5/1  "<Mz>"
  Reshape3/1 -> Matrix Concatenate/1
  Reshape4/1 -> Matrix Concatenate/2
  Reshape5/1 -> Matrix Concatenate/3
  Matrix Concatenate/1 -> M/1  "M"
  Reshape/1 -> z/1  "z"

== system CAVE_MachE_sil_test_v2/Vehicle Under Test/Vehicle/Vehicle Dynamics/Vehicle 14DOF/Suspension/MacPherson Front Suspension Solid Axle Rear Suspension/Steer Rate Adapter ==
  Veh : Inport
  Add : Sum
  Bus Selector3 : BusSelector  OutputSignals=BdyFrm.Cg.AngVel.r
  Constant : Constant  Value=zeros(1,4)
  Matrix Concatenate : Concatenate  NumInputs=3  Mode=Multidimensional array
  Matrix Concatenate1 : Concatenate  NumInputs=3  Mode=Multidimensional array
  Reshape2 : Reshape  OutputDimensionality=Row vector (2-D)
  Reshape3 : Reshape  OutputDimensionality=Row vector (2-D)
  Reshape4 : Reshape  OutputDimensionality=Row vector (2-D)
  Selector3 : Selector  InputPortWidth=1  IndexOptions=Index vector (dialog)  Indices=[1 1 1 1]  OutputSizes=1
  SteerRates : Constant  Value=zeros(1,4)
  AngVel : Outport  VectorParamsAs1DForOutWhenUnconnected=off
  wires:
  Reshape2/1 -> Matrix Concatenate1/1, Matrix Concatenate1/3, Matrix Concatenate1/2
  Constant/1 -> Reshape3/1
  Selector3/1 -> Reshape4/1
  Bus Selector3/1 -> Selector3/1  "<r>"
  Matrix Concatenate/1 -> Add/2
  SteerRates/1 -> Reshape2/1
  Reshape4/1 -> Matrix Concatenate/3
  Reshape3/1 -> Matrix Concatenate/2, Matrix Concatenate/1
  Matrix Concatenate1/1 -> Add/1
  Veh/1 -> Bus Selector3/1
  Add/1 -> AngVel/1  "AngVel"

== system CAVE_MachE_sil_test_v2/Vehicle Under Test/Vehicle/Vehicle Dynamics/Vehicle 14DOF/Suspension/MacPherson Front Suspension Solid Axle Rear Suspension/Steering Adapter ==
  Steer : Inport
  Reshape1 : Reshape  OutputDimensionality=Row vector (2-D)
  Selector : Selector  IndexOptions=Index vector (dialog)  Indices=[1 2]  OutputSizes=1
  StrgAng : Outport  VectorParamsAs1DForOutWhenUnconnected=off
  wires:
  Reshape1/1 -> StrgAng/1
  Steer/1 -> Selector/1
  Selector/1 -> Reshape1/1

== system CAVE_MachE_sil_test_v2/Vehicle Under Test/Vehicle/Vehicle Dynamics/Vehicle 14DOF/Suspension/MacPherson Front Suspension Solid Axle Rear Suspension/Vehicle Adapter ==
  Veh : Inport
  Bus Creator3 : BusCreator  Inputs=2
  Bus Selector1 : BusSelector  OutputSignals=InertFrm.FrntAxl.Lft.Disp.X,InertFrm.FrntAxl.Lft.Disp.Y,InertFrm.FrntAxl.Lft.Disp.Z,InertFrm.FrntAxl.Rght.Disp.X,InertFrm.FrntAxl.Rght.Disp.Y,InertFrm.FrntAxl.Rght.Disp.Z,InertFrm.RearAxl.Lft.Disp.X,InertFrm.RearAxl.Lft.Disp.Y,InertFrm.RearAxl.Lft.Disp.Z,InertFrm.RearAxl.Rght.Disp.X,InertFrm.RearAxl.Rght.Disp.Y,InertFrm.RearAxl.Rght.Disp.Z
  Bus Selector2 : BusSelector  OutputSignals=BdyFrm.FrntAxl.Lft.Vel.xdot,BdyFrm.FrntAxl.Lft.Vel.ydot,BdyFrm.FrntAxl.Lft.Vel.zdot,BdyFrm.FrntAxl.Rght.Vel.xdot,BdyFrm.FrntAxl.Rght.Vel.ydot,BdyFrm.FrntAxl.Rght.Vel.zdot,BdyFrm.RearAxl.Lft.Vel.xdot,BdyFrm.RearAxl.Lft.Vel.ydot,BdyFrm.RearAxl.Lft.Vel.zdot,BdyFrm.RearAxl.Rght.Vel.xdot,BdyFrm.RearAxl.Rght.Vel.ydot,BdyFrm.RearAxl.Rght.Vel.zdot
  Inertial Frame CG to Axle Offset : Constant  Value=[zeros(2,4);0.134*ones(1,4)]
  Mux1 : Mux  Inputs=12
  Mux2 : Mux  Inputs=12
  Reshape : Reshape  OutputDimensionality=Customize  OutputDimensions=[3,4]
  Reshape2 : Reshape  OutputDimensionality=Customize  OutputDimensions=[3,4]
  Sum : Sum  Inputs=|+-
  VehSusp : Outport  VectorParamsAs1DForOutWhenUnconnected=off
  wires:
  Veh/1 -> Bus Selector2/1, Bus Selector1/1
  Reshape2/1 -> Bus Creator3/2  "V"
  Bus Creator3/1 -> VehSusp/1  "Veh"
  Reshape/1 -> Sum/1
  Bus Selector1/1 -> Mux2/1  "<X>"
  Bus Selector1/2 -> Mux2/2  "<Y>"
  Bus Selector1/3 -> Mux2/3  "<Z>"
  Bus Selector1/4 -> Mux2/4  "<X>"
  Bus Selector1/5 -> Mux2/5  "<Y>"
  Bus Selector1/6 -> Mux2/6  "<Z>"
  Bus Selector1/7 -> Mux2/7  "<X>"
  Bus Selector1/8 -> Mux2/8  "<Y>"
  Bus Selector1/9 -> Mux2/9  "<Z>"
  Bus Selector1/10 -> Mux2/10  "<X>"
  Bus Selector1/11 -> Mux2/11  "<Y>"
  Bus Selector1/12 -> Mux2/12  "<Z>"
  Bus Selector2/1 -> Mux1/1  "<xdot>"
  Bus Selector2/2 -> Mux1/2  "<ydot>"
  Bus Selector2/3 -> Mux1/3  "<zdot>"
  Bus Selector2/4 -> Mux1/4  "<xdot>"
  Bus Selector2/5 -> Mux1/5  "<ydot>"
  Bus Selector2/6 -> Mux1/6  "<zdot>"
  Bus Selector2/7 -> Mux1/7  "<xdot>"
  Bus Selector2/8 -> Mux1/8  "<ydot>"
  Bus Selector2/9 -> Mux1/9  "<zdot>"
  Bus Selector2/10 -> Mux1/10  "<xdot>"
  Bus Selector2/11 -> Mux1/11  "<ydot>"
  Bus Selector2/12 -> Mux1/12  "<zdot>"
  Mux1/1 -> Reshape2/1
  Mux2/1 -> Reshape/1
  Inertial Frame CG to Axle Offset/1 -> Sum/2
  Sum/1 -> Bus Creator3/1  "P"

== system CAVE_MachE_sil_test_v2/Vehicle Under Test/Vehicle/Vehicle Dynamics/Vehicle 14DOF/Suspension/MacPherson Front Suspension Solid Axle Rear Suspension/Wheel  Adapter ==
  Wheels : Inport
  Bus Selector : BusSelector  OutputSignals=TireFrame.Fx,TireFrame.Fy
  Bus Selector1 : BusSelector  OutputSignals=TireFrame.Re
  Bus Selector2 : BusSelector  OutputSignals=TireFrame.Mx,TireFrame.My,TireFrame.Mz
  Bus Selector3 : BusSelector  OutputSignals=TireFrame.z,TireFrame.zdot
  Matrix Concatenate : Concatenate  NumInputs=3  Mode=Multidimensional array
  Reshape{,1..7} (8 alike) : Reshape  OutputDimensionality=Row vector (2-D)
  WhlFx : Outport  VectorParamsAs1DForOutWhenUnconnected=off
  WhlFy : Outport  Port=2  VectorParamsAs1DForOutWhenUnconnected=off
  z : Outport  Port=3  VectorParamsAs1DForOutWhenUnconnected=off
  zdot : Outport  Port=4  VectorParamsAs1DForOutWhenUnconnected=off
  M : Outport  Port=5  VectorParamsAs1DForOutWhenUnconnected=off
  Re : Outport  Port=6  VectorParamsAs1DForOutWhenUnconnected=off
  wires:
  Reshape7/1 -> WhlFy/1
  Reshape6/1 -> WhlFx/1
  Bus Selector/1 -> Reshape6/1  "<Fx>"
  Bus Selector/2 -> Reshape7/1  "<Fy>"
  Bus Selector3/1 -> Reshape/1  "<z>"
  Wheels/1 -> Bus Selector1/1, Bus Selector2/1, Bus Selector3/1, Bus Selector/1
  Bus Selector3/2 -> Reshape2/1  "<zdot>"
  Reshape2/1 -> zdot/1  "zdot"
  Bus Selector1/1 -> Reshape1/1  "<Re>"
  Reshape1/1 -> Re/1  "Re"
  Bus Selector2/1 -> Reshape3/1  "<Mx>"
  Bus Selector2/2 -> Reshape4/1  "<My>"
  Bus Selector2/3 -> Reshape5/1  "<Mz>"
  Reshape3/1 -> Matrix Concatenate/1
  Reshape4/1 -> Matrix Concatenate/2
  Reshape5/1 -> Matrix Concatenate/3
  Matrix Concatenate/1 -> M/1  "M"
  Reshape/1 -> z/1  "z"

== system CAVE_MachE_sil_test_v2/Vehicle Under Test/Vehicle/Vehicle Dynamics/Vehicle 14DOF/Suspension/MacPherson Suspension/Steer Rate Adapter ==
  Veh : Inport
  Add : Sum
  Bus Selector3 : BusSelector  OutputSignals=BdyFrm.Cg.AngVel.r
  Constant : Constant  Value=zeros(1,4)
  Matrix Concatenate : Concatenate  NumInputs=3  Mode=Multidimensional array
  Matrix Concatenate1 : Concatenate  NumInputs=3  Mode=Multidimensional array
  Reshape2 : Reshape  OutputDimensionality=Row vector (2-D)
  Reshape3 : Reshape  OutputDimensionality=Row vector (2-D)
  Reshape4 : Reshape  OutputDimensionality=Row vector (2-D)
  Selector3 : Selector  InputPortWidth=1  IndexOptions=Index vector (dialog)  Indices=[1 1 1 1]  OutputSizes=1
  SteerRates : Constant  Value=zeros(1,4)
  AngVel : Outport  VectorParamsAs1DForOutWhenUnconnected=off
  wires:
  Reshape2/1 -> Matrix Concatenate1/1, Matrix Concatenate1/3, Matrix Concatenate1/2
  Constant/1 -> Reshape3/1
  Selector3/1 -> Reshape4/1
  Bus Selector3/1 -> Selector3/1  "<r>"
  Matrix Concatenate/1 -> Add/2
  SteerRates/1 -> Reshape2/1
  Reshape4/1 -> Matrix Concatenate/3
  Reshape3/1 -> Matrix Concatenate/2, Matrix Concatenate/1
  Matrix Concatenate1/1 -> Add/1
  Veh/1 -> Bus Selector3/1
  Add/1 -> AngVel/1  "AngVel"

== system CAVE_MachE_sil_test_v2/Vehicle Under Test/Vehicle/Vehicle Dynamics/Vehicle 14DOF/Suspension/MacPherson Suspension/Steering Adapter ==
  Steer : Inport
  Reshape1 : Reshape  OutputDimensionality=Row vector (2-D)
  Selector : Selector  IndexOptions=Index vector (dialog)  Indices=[1 2]  OutputSizes=1
  StrgAng : Outport  VectorParamsAs1DForOutWhenUnconnected=off
  wires:
  Reshape1/1 -> StrgAng/1
  Steer/1 -> Selector/1
  Selector/1 -> Reshape1/1
